simulink model "SIL1"  (R2024b)
settings: Solver=VariableStepAuto  StartTime=0.0  StopTime=10.0  RelTol=1e-3
values from neighbouring files (symbols this model uses):
  b = 7.2e-5    (= 7.2e-05)    [HIL.m]    (also in SIL.m = 4.2697318139e-06)
  Cr = 0    [SIL.m]
  Fs = 0    [SIL.m]
  J = 6.87e-5    (= 6.87e-05)    [HIL.m]    (also in SIL.m = 4.14e-06)
  Kc = Ke    (= 0.0241)    [HIL.m]    (also in SIL.m)
  Ke = 24.1e-3    (= 0.0241)    [HIL.m]    (also in SIL.m = 0.024114385317)
  L = 0.42e-3    (= 0.00042)    [HIL.m]    (also in SIL.m)
  R = 2.99    [HIL.m]    (also in SIL.m)
settings Model: Creator=tclaverie303  LastModifiedBy=tclaverie303

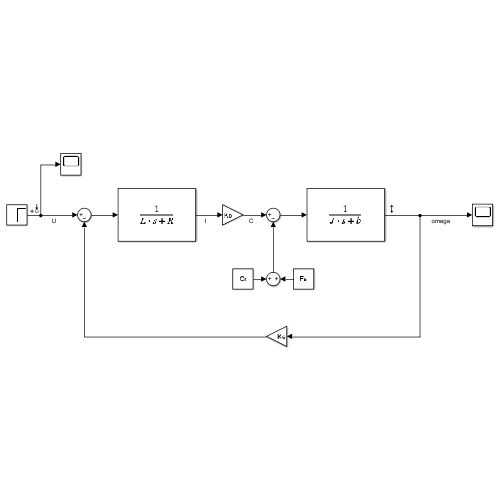
[thumbnail: Simulink's stored preview of the top-level diagram]
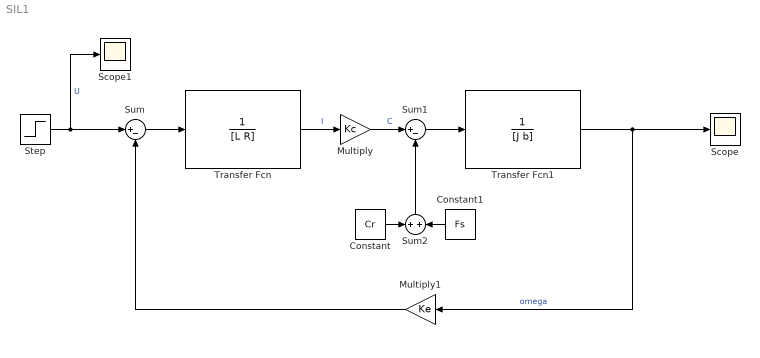
== system SIL1 ==
  Constant : Constant  Value=Cr
  Constant1 : Constant  Value=Fs
  Multiply : Gain  Gain=Kc
  Multiply1 : Gain  Gain=Ke
  Scope : Scope
  Scope1 : Scope
  Step : Step  After=12  SampleTime=0
  Sum : Sum  Inputs=|+-
  Sum1 : Sum  Inputs=|+-
  Sum2 : Sum
  Transfer Fcn : TransferFcn  Denominator=[L R]
  Transfer Fcn1 : TransferFcn  Denominator=[J b]
  wires:
  Step/1 -> Scope1/1, Sum/1  "U"
  Sum/1 -> Transfer Fcn/1
  Transfer Fcn/1 -> Multiply/1  "I"
  Multiply/1 -> Sum1/1  "C"
  Sum1/1 -> Transfer Fcn1/1
  Constant/1 -> Sum2/1
  Constant1/1 -> Sum2/2
  Sum2/1 -> Sum1/2
  Multiply1/1 -> Sum/2
  Transfer Fcn1/1 -> Multiply1/1, Scope/1  "omega"
